simulink model "BEVplantModel"  (R2022b)
settings: Solver=daessc  StartTime=0  StopTime=50  RelTol=1e-3
PreLoadFcn:
  | % Load all parameters
  | BEVplantModelParam;
undefined symbols (not defined in the file): battery, cabin_T_init, coolant_pipe_D, coolant_valve_D_ratio_max, coolant_valve_D_ratio_min, coolant_valve_displacement, electricDrive, max_torque, vehicle, vehicleThermal
libraries: fl_lib x292, nesl_utility x67, SimscapeFluids_lib x15, ee_lib x11, sdl_lib x8, BatteryCurrentManagement x3, slpidlib x3, simulink x2, BatteryThermalManagement x1, autolibshared x1
(part 10 of 10)

== system BEVplantModel/Vehicle/Front Motor (EM1)/Emotor/Temperature/Stator Thermal Block/Loss Correction ==
  PS Add : fl_lib/Physical Signals/Functions/PS Add
  PS Product : fl_lib/Physical Signals/Functions/PS Product
  PS Subtract : fl_lib/Physical Signals/Functions/PS Subtract
  Ref Temp Of loss calculations : fl_lib/Physical Signals/Sources/PS Constant  constant=298 K
  add 1 : fl_lib/Physical Signals/Sources/PS Constant  constant=1
  joule coefficient : fl_lib/Physical Signals/Functions/PS Gain  gain=0.00386 1/K
  Temp : PMIOPort  Side=Left
  I2R_Loss : PMIOPort  Port=2  Side=Left
  HCorrect : PMIOPort  Port=3  Side=Right
  connections:
  add 1/RConn1 -- PS Add/LConn2
  Ref Temp Of loss calculations/RConn1 -- PS Subtract/LConn2
  Temp/RConn1 -- PS Subtract/LConn1
  I2R_Loss/RConn1 -- PS Product/LConn2
  PS Add/RConn1 -- PS Product/LConn1
  joule coefficient/RConn1 -- PS Add/LConn1
  PS Subtract/RConn1 -- joule coefficient/LConn1
  HCorrect/RConn1 -- PS Product/RConn1

== system BEVplantModel/Vehicle/Rear Motor (EM2)/Emotor/Temperature/Stator Thermal Block/Loss Correction ==
  PS Add : fl_lib/Physical Signals/Functions/PS Add
  PS Product : fl_lib/Physical Signals/Functions/PS Product
  PS Subtract : fl_lib/Physical Signals/Functions/PS Subtract
  Ref Temp Of loss calculations : fl_lib/Physical Signals/Sources/PS Constant  constant=298 K
  add 1 : fl_lib/Physical Signals/Sources/PS Constant  constant=1
  joule coefficient : fl_lib/Physical Signals/Functions/PS Gain  gain=0.00386 1/K
  Temp : PMIOPort  Side=Left
  I2R_Loss : PMIOPort  Port=2  Side=Left
  HCorrect : PMIOPort  Port=3  Side=Right
  connections:
  add 1/RConn1 -- PS Add/LConn2
  Ref Temp Of loss calculations/RConn1 -- PS Subtract/LConn2
  Temp/RConn1 -- PS Subtract/LConn1
  I2R_Loss/RConn1 -- PS Product/LConn2
  PS Add/RConn1 -- PS Product/LConn1
  joule coefficient/RConn1 -- PS Add/LConn1
  PS Subtract/RConn1 -- joule coefficient/LConn1
  HCorrect/RConn1 -- PS Product/RConn1

== stateflow chart BEVplantModel/Controller/Vehicle Control/Torque Control/Trq Split Fac/Stateflow ==
  state FrontWheel
    Mode=0;
    TrqEm1Fac=1;
    TrqEm2Fac=0;
  state BrakeDistr
    Mode=2;
    TrqEm1Fac=1;
  state AWD
    Mode=1;
    TrqEm1Fac=0.6;
    TrqEm2Fac=0.4;
  (default) -> FrontWheel
  FrontWheel -> BrakeDistr [order 2] : [Tq<=0]
  BrakeDistr -> FrontWheel : [Tq>0]
  AWD -> FrontWheel : [Tq<10]
  FrontWheel -> AWD [order 1] : [Tq>180]
  data: Tq input; Mode output; TrqEm2Fac output; TrqEm1Fac output

== stateflow chart BEVplantModel/Controller/BMS/Battery Protection Logic/State Flow/Fault Protection ==
  state BatteryRequest [parallel]
    settings: executionOrder=1
    state BatteryConnect_Req
      BatReq=1;
    state BatteryDischarging
      BatSt=3;
    state Standby
      BatSt=0;
    state OpenDchg
      RelDchgOpening=1;
    state BatteryDchgReq
      BatReq=3;
      RelDchgClosing=1;
    state Battery_Connect
      Rclosing=1;
    state Idle_State
      BatSt=1;
    state OpenChg
      RelChgOpening=1;
    state Battery_disconnect
      BatReq=0;
      Ropening=1;
    state BatteryChgReq
      BatReq=2;
      RelChgClosing=1;
    state BatteryCharging
      BatSt=2;
    (default) -> Standby : {BatReq=0;Rpos=0; Rneg=0;
        |  Rclosing=0;Ropening=0;
        | RelChgOpening=0;RelChgClosing=0;
        | RelDchgOpening=0;RelDchgClosing=0;}
    BatteryDischarging -> BatteryConnect_Req : [BatCmd~=3 || BatSoC.Min<0.01 || FaultDet==1]
    BatteryConnect_Req -> OpenDchg [order 2] : [BatSt==3]
    Standby -> BatteryConnect_Req : [BatCmd~=0 && BatSoC.Min>=0.05 ...
        | && FaultDet==0 && CountFault==0]
    OpenDchg -> Idle_State : [RelDchgClose==0]
    Battery_disconnect -> Standby : [Rclose==0]
    BatteryDchgReq -> BatteryDischarging : [RelDchgClose==1]
    Idle_State -> BatteryDchgReq [order 1] : [BatCmd==3 && FaultDet==0 ...
        | &&  BatSoC.Min>=0.05]
    BatteryConnect_Req -> Battery_Connect [order 1] : [ FaultDet==0 ...
        | && CountFault==0 ...
        | && BatSt==0]
    Battery_Connect -> Idle_State : [Rclose==1]
    BatteryCharging -> BatteryConnect_Req : [BatCmd~=2 || BatSoC.Max>0.99 ...
        | || FaultDet==1]
    BatteryConnect_Req -> (junction 399) [order 3] : [BatSt==2]
    (junction 399) -> OpenChg
    Idle_State -> (junction 392) [order 2] : [BatCmd==0 || BatSoC.Min<=0.01 ...
        |  || BatSoC.Min>=0.99 || FaultDet==1]
    OpenChg -> Idle_State : [RelChgClose==0]
    (junction 392) -> (junction 393)
    Idle_State -> BatteryChgReq [order 3] : [BatCmd==2 ...
        | && BatSoC.Max<=0.97 ...
        |  && FaultDet==0 ]
    (junction 394) -> Battery_disconnect
    BatteryChgReq -> (junction 113) : [RelChgClose==1]
    (junction 113) -> BatteryCharging
    (junction 393) -> (junction 394)
  state Protection [group]
    state ThermalFault [parallel]
      settings: executionOrder=1
      state NoFault
      state DebounceMin
      state FaultDetected
        FaultDet=1;
        FaultDisp.ThermFault=1;
      state DebounceMax
      (default) -> NoFault : {FaultDet=0;
          | FaultTh.Min=0;
          | FaultTh.Max=0;
          | ThermFault=0;}
      DebounceMin -> NoFault [order 1] : [Tp.Min>MinThLmt]
      NoFault -> DebounceMin [order 1] : [Tp.Min<MinThLmt ...
          | && Rclose==1]
      DebounceMin -> FaultDetected [order 2] : after(10,sec)
          | {FaultTh.Min=1;}
      NoFault -> DebounceMax [order 2] : [Tp.Max>MaxThLmt ...
          | && Rclose==1]
      DebounceMax -> FaultDetected [order 2] : after(10,sec)
          | {FaultTh.Max=1;}
      DebounceMax -> NoFault [order 1] : [Tp.Max<MaxThLmt]
    state CurrFault [parallel]
      settings: executionOrder=4
    state VoltageFault [parallel]
      settings: executionOrder=3
    state Reset [parallel]
      settings: executionOrder=2
      state Reset
        CountFault=0;
        VoltFault=0;
        ElecFault=0;
        FaultDet=0;
        FaultDisp.VoltFault=0;
        FaultDisp.CountMin=0;CountMin=0;
        FaultDisp.CountMax=0;CountMax=0;
        FaultDisp.CurrFault=0;
        FaultDisp.CountCh=0;CountCh=0;
        FaultDisp.CountDch=0;CountDch=0;
      state Wait
      (default) -> Wait
      Wait -> Protection.Reset.Reset : [FaultReset==1]
      Protection.Reset.Reset -> Wait : [FaultReset==0]
  state RelayOperationBattery [parallel]
    settings: executionOrder=2
    state RelayOpen
      state PosRelayOpen
        Rpos=0;
      state NegRelayOpen
        Rneg=0;
      state Opened
        Rclose=0;
        Ropening=0;
      (default) -> PosRelayOpen
      PosRelayOpen -> NegRelayOpen : after(100,msec)
      NegRelayOpen -> Opened : after(100,msec)
    state RelayClose
      state NegRelayClose
        Rneg=1;
        Rclose=0;
      state PosRelayClose
        Rpos=1;
      state Closed
        Rclose=1;
        Rclosing=0;
      (default) -> NegRelayClose
      NegRelayClose -> PosRelayClose : after(100,msec)
      PosRelayClose -> Closed : after(100,msec)
    (default) -> RelayOpen : {Rneg=0; Rpos=0;
        | Rclose=0;}
    Opened -> RelayClose : [Rclosing==1]
    Closed -> RelayOpen : [Ropening==1]
  state Relay_Discharge [parallel]
    settings: executionOrder=3
  state Relay_Charge [parallel]
    settings: executionOrder=4
  data: Count1 function_output; Value2 function_input; Count2 function_output; ElecFlag function_output; ElecFault function_output; CountFault function_output; Rclose function_output; ThermFault function_output; Lmt2 function_input; Lmt1 function_input; Value1 function_input; FaultPath1 function_output; FaultPath2 function_output; offset function_input; Count1 function_output; Value2 function_input; Count2 function_output; ElecFlag function_output; ElecFault function_output; CountFault function_output; Rclose function_output; ThermFault function_output; Lmt2 function_input; Lmt1 function_input; Value1 function_input; FaultPath1 function_output; FaultPath2 function_output; offset function_input; RelClosing function_output; RelClose function_output; RelOpening function_output; RelClosing function_output; RelClose function_output; RelOpening function_output; I input Bus: I_Current; FaultDet output double =0; FaultElec output Bus: I_Current; CurLmt input Bus: I_Current; Volt input Bus: CellVoltage; Rclosing local double; Ropening local double; FaultTh output Bus: MaxMinLimit; Tp input Bus: MaxMinLimit; BatSt output double; BatReq local; BatSoC input Bus: MaxMinLimit; BatCmd input; Rpos output double; Rneg output double; FaultVolt output Bus: MaxMinLimit; CountFault local double; ThermFault local double; CountCh local double; CountDch local double; CountMax local double; CountMin local double; FaultDisp output Bus: FaultDisp; ElecFault local double =0; VoltFault local double; FaultReset input double; RelChg output double; RelDchg output double; RelChgClosing local double; RelChgOpening local double; RelDchgClosing local double; RelDchgOpening local double; RelDchgClose local double; RelChgClose local double; Rclose local double; MaxVoltLmt parameter double; MinVoltLmt parameter double; MaxThLmt parameter double; MinThLmt parameter double; CurrOffset parameter double; VoltOffset parameter double

== stateflow chart BEVplantModel/Controller/BMS/Battery Protection Logic/State Flow/Fault Protection/Protection.CurrFault ==
  state FaultDetected
    en,du:
    FaultDet=1;
    ElecFlag=1;
    ElecFault = ...
    duration(ElecFlag==1 ...
    ,msec);
  state NoFault
    en:
    ElecFault=0;
    ElecFlag=0;
  state DebouncePath1
  state FaultCounter
  state DebouncePath2
  (default) -> NoFault : {Count1=0;
      | Count2=0;
      | CountFault=0;
      | FaultPath1=0;
      | FaultPath2=0;
      | FaultDet=0;}
  NoFault -> DebouncePath1 [order 1] : [Value1<Lmt1-offset && Rclose==1]
  DebouncePath1 -> FaultDetected : after(1,sec)
      | {FaultPath1=1;
      | Count1=Count1+1;}
  NoFault -> DebouncePath1 [order 3] : [duration(Value1<Lmt1)>1 ...
      | && Rclose==1]
  FaultCounter -> NoFault [order 1] : [Count1==5 || Count2==5]
      | {CountFault=1;}
  FaultDetected -> FaultCounter : [Rclose==0 ...
      |  && ThermFault==0 ...
      | && ElecFault>=1000]
  FaultCounter -> NoFault [order 2] : {FaultPath1=0;
      | FaultPath2=0;FaultDet=0;}
  NoFault -> DebouncePath2 [order 4] : [duration(Value2>Lmt2)>1 ...
      | && Rclose==1]
  DebouncePath2 -> FaultDetected : after(1,sec)
      | {FaultPath2=1;
      | Count2=Count2+1;}
  NoFault -> DebouncePath2 [order 2] : [Value2>Lmt2+offset && Rclose==1]
  data: FaultDet output double =0; Count1 output double; Count2 output double; ElecFlag output double =0; ElecFault output double =0; CountFault output double; Rclose output double; ThermFault output double; Value2 input; Lmt2 input; Lmt1 input; Value1 input; FaultPath1 output; FaultPath2 output; offset input double

== stateflow chart BEVplantModel/Controller/BMS/Battery Protection Logic/State Flow/Fault Protection/Protection.VoltageFault ==
  state FaultDetected
    en,du:
    FaultDet=1;
    ElecFlag=1;
    ElecFault = ...
    duration(ElecFlag==1 ...
    ,msec);
  state NoFault
    en:
    ElecFault=0;
    ElecFlag=0;
  state DebouncePath1
  state FaultCounter
  state DebouncePath2
  (default) -> NoFault : {Count1=0;
      | Count2=0;
      | CountFault=0;
      | FaultPath1=0;
      | FaultPath2=0;
      | FaultDet=0;}
  NoFault -> DebouncePath1 [order 1] : [Value1<Lmt1-offset && Rclose==1]
  DebouncePath1 -> FaultDetected : after(1,sec)
      | {FaultPath1=1;
      | Count1=Count1+1;}
  NoFault -> DebouncePath1 [order 3] : [duration(Value1<Lmt1)>1 ...
      | && Rclose==1]
  FaultCounter -> NoFault [order 1] : [Count1==5 || Count2==5]
      | {CountFault=1;}
  FaultDetected -> FaultCounter : [Rclose==0 ...
      |  && ThermFault==0 ...
      | && ElecFault>=1000]
  FaultCounter -> NoFault [order 2] : {FaultPath1=0;
      | FaultPath2=0;FaultDet=0;}
  NoFault -> DebouncePath2 [order 4] : [duration(Value2>Lmt2)>1 ...
      | && Rclose==1]
  DebouncePath2 -> FaultDetected : after(1,sec)
      | {FaultPath2=1;
      | Count2=Count2+1;}
  NoFault -> DebouncePath2 [order 2] : [Value2>Lmt2+offset && Rclose==1]
  data: FaultDet output double =0; Count1 output double; Count2 output double; ElecFlag output double =0; ElecFault output double =0; CountFault output double; Rclose output double; ThermFault output double; Value2 input; Lmt2 input; Lmt1 input; Value1 input; FaultPath1 output; FaultPath2 output; offset input double

== stateflow chart BEVplantModel/Controller/BMS/Battery Protection Logic/State Flow/Fault Protection/Relay_Charge ==
  state RelayOpen
    state RelayOpen
      Relay=0;
    state Opened
      RelClose=0;
      RelOpening=0;
    (default) -> RelayOpen.RelayOpen
    RelayOpen.RelayOpen -> Opened : after(100,msec)
  state RelayClose
    state PosRelayClose
      Relay=1;
    state Closed
      RelClose=1;
      RelClosing=0;
    (default) -> PosRelayClose
    PosRelayClose -> Closed : after(100,msec)
  (default) -> RelayOpen : {RelClose=0;Relay=0;}
  Opened -> RelayClose : [RelClosing==1]
  Closed -> RelayOpen : [RelOpening==1]
  data: RelClosing output; RelClose output; Relay output; RelOpening output

== stateflow chart BEVplantModel/Controller/BMS/Battery Protection Logic/State Flow/Fault Protection/Relay_Discharge ==
  state RelayOpen
    state RelayOpen
      Relay=0;
    state Opened
      RelClose=0;
      RelOpening=0;
    (default) -> RelayOpen.RelayOpen
    RelayOpen.RelayOpen -> Opened : after(100,msec)
  state RelayClose
    state PosRelayClose
      Relay=1;
    state Closed
      RelClose=1;
      RelClosing=0;
    (default) -> PosRelayClose
    PosRelayClose -> Closed : after(100,msec)
  (default) -> RelayOpen : {RelClose=0;Relay=0;}
  Opened -> RelayClose : [RelClosing==1]
  Closed -> RelayOpen : [RelOpening==1]
  data: RelClosing output; RelClose output; Relay output; RelOpening output
